simulink model "WCS_Simulink"  (Simulink 8.1)
settings: Solver=ode4  StartTime=0.0  StopTime=Tf  FixedStep=delta_t  RelTol=1e-3
values from neighbouring files (symbols this model uses):
  A = [-3 0;0 0.2]    [Linear_WCS_main.m]
  B = [1; 1]    [Linear_WCS_main.m]
  C = [1 1]    [Linear_WCS_main.m]
  delta_t = 1/sensor_sampling_rate    (= 0.2)    [Linear_WCS_main.m]
  T = [1 1;0 1]    [Linear_WCS_main.m]
  uini = 0    [Linear_WCS_main.m]
  Xini = [x1ini;x2ini]    [Linear_WCS_main.m]
  Xsp = [x1sp;x2sp]    [Linear_WCS_main.m]
settings Model: Creator=Rhine  LastModifiedBy=yehanspc

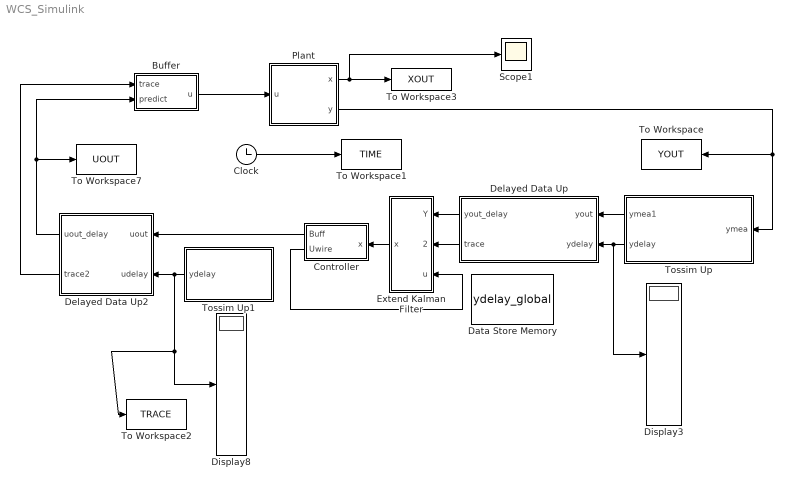
== system WCS_Simulink ==
  Buffer : Subsystem
  Clock : Clock
  Controller : Subsystem
  Data Store Memory : DataStoreMemory  DataStoreName=ydelay_global  ReadBeforeWriteMsg=warning  WriteAfterWriteMsg=warning  WriteAfterReadMsg=warning  InitialValue=[1; 1; 1; 1; 1; 1; 1; 1; 1; 1; 1; 1; 1; 1; 1]  OutDataTypeStr=uint32
  Delayed Data Up : MATLAB Function  TreatAsAtomicUnit=on
  Delayed Data Up2 : MATLAB Function  TreatAsAtomicUnit=on
  Display3 : Display
  Display8 : Display
  Extend Kalman Filter : Subsystem
  Plant : Subsystem
  Scope1 : Scope
  To Workspace : ToWorkspace  VariableName=YOUT  SampleTime=-1
  To Workspace1 : ToWorkspace  VariableName=TIME  SampleTime=-1
  To Workspace2 : ToWorkspace  VariableName=TRACE  SampleTime=-1
  To Workspace3 : ToWorkspace  VariableName=XOUT  SampleTime=-1
  To Workspace7 : ToWorkspace  VariableName=UOUT  SampleTime=-1
  Tossim Up : MATLAB Function  TreatAsAtomicUnit=on
  Tossim Up1 : MATLAB Function  TreatAsAtomicUnit=on
  wires:
  Clock/1 -> To Workspace1/1
  Tossim Up/1(ymea1) -> Delayed Data Up/1(yout)
  Tossim Up/2(ydelay) -> Display3/1, Delayed Data Up/2(ydelay)
  Plant/2(y) -> Tossim Up/1(ymea), To Workspace/1
  Tossim Up1/1(ydelay) -> Delayed Data Up2/2(udelay), To Workspace2/1, Display8/1
  Controller/2(Uwire) -> Extend Kalman Filter/3(u)
  Delayed Data Up/1(yout_delay) -> Extend Kalman Filter/1(Y)
  Extend Kalman Filter/1(x) -> Controller/1(x)
  Plant/1(x) -> Scope1/1, To Workspace3/1
  Delayed Data Up/2(trace) -> Extend Kalman Filter/2("trace ")
  Delayed Data Up2/2(trace2) -> Buffer/1(trace)
  Delayed Data Up2/1(uout_delay) -> Buffer/2(predict), To Workspace7/1
  Controller/1(Buff) -> Delayed Data Up2/1(uout)
  Buffer/1(u) -> Plant/1(u)

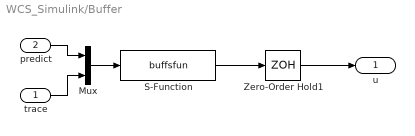
== system WCS_Simulink/Buffer ==
  trace : Inport
  predict : Inport  Port=2
  Mux : Mux  Inputs=2
  S-Function : S-Function  FunctionName=buffsfun  EnableBusSupport=off
  Zero-Order Hold1 : ZeroOrderHold  SampleTime=delta_t
  u : Outport
  wires:
  S-Function/1 -> Zero-Order Hold1/1
  Zero-Order Hold1/1 -> u/1
  Mux/1 -> S-Function/1
  predict/1 -> Mux/1
  trace/1 -> Mux/2

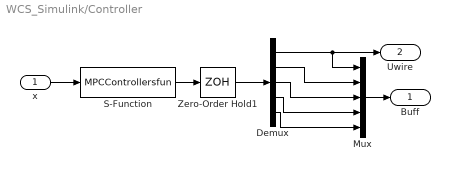
== system WCS_Simulink/Controller ==
  x : Inport
  Demux : Demux  Outputs=5
  Mux : Mux  Inputs=5
  S-Function : S-Function  FunctionName=MPCControllersfun  Parameters=A,B,C,T,uini,Xsp,delta_t  EnableBusSupport=off
  Zero-Order Hold1 : ZeroOrderHold  SampleTime=delta_t
  Buff : Outport
  Uwire : Outport  Port=2
  wires:
  x/1 -> S-Function/1
  S-Function/1 -> Zero-Order Hold1/1
  Zero-Order Hold1/1 -> Demux/1
  Demux/1 -> Mux/1, Uwire/1
  Mux/1 -> Buff/1
  Demux/2 -> Mux/2
  Demux/3 -> Mux/3
  Demux/4 -> Mux/4
  Demux/5 -> Mux/5

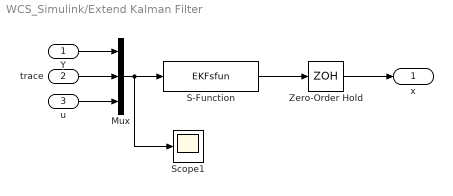
== system WCS_Simulink/Extend Kalman Filter ==
  Y : Inport
  "trace " : Inport  Port=2
  u : Inport  Port=3
  Mux : Mux  Inputs=3
  S-Function : S-Function  FunctionName=EKFsfun  Parameters=A,B,C,T,delta_t  EnableBusSupport=off
  Scope1 : Scope
      settings: SaveName=ScopeData2
  Zero-Order Hold : ZeroOrderHold  SampleTime=delta_t
  x : Outport
  wires:
  Y/1 -> Mux/1
  Mux/1 -> Scope1/1, S-Function/1
  u/1 -> Mux/3
  S-Function/1 -> Zero-Order Hold/1
  Zero-Order Hold/1 -> x/1
  "trace "/1 -> Mux/2

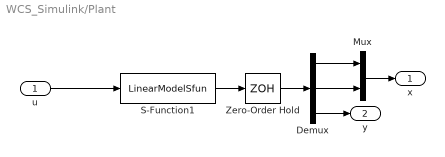
== system WCS_Simulink/Plant ==
  u : Inport
  Demux : Demux  Outputs=3
  Mux : Mux  Inputs=2
  S-Function1 : S-Function  FunctionName=LinearModelSfun  Parameters=A,B,C,T,Xini  EnableBusSupport=off
  Zero-Order Hold : ZeroOrderHold  SampleTime=delta_t
  x : Outport
  y : Outport  Port=2
  wires:
  S-Function1/1 -> Zero-Order Hold/1
  u/1 -> S-Function1/1
  Zero-Order Hold/1 -> Demux/1
  Demux/1 -> Mux/1
  Demux/2 -> Mux/2
  Mux/1 -> x/1
  Demux/3 -> y/1

== matlab function Tossim Up ==
  data: ymea1 output double; ymea input double; ydelay output double; ydelay_global data_store_memory double
function [ymea1, ydelay]  = Tossim_block(ymea)
% Inputs:
% ymea: measurement from structure
% Outputs:
% ymea1: measurement output
% ydelay: delay traces
persistent delay1 % delay trace
persistent i  % count
global ydelay_global


% allow these matlab functions to be used in Embedded Matlab block
eml.extrinsic('python');
eml.extrinsic('num2str');
eml.extrinsic('str2num');
eml.extrinsic('delay_summary');
eml.extrinsic('disp');
eml.extrinsic('ps_aggregation');
eml.extrinsic('for');
eml.extrinsic('end');

if isempty(i)
    i = 0;
end

ydelay = [1 0 0 0 0 0 0 0 0]';
% call python to communicate with TOSSIM

call_count = 18; %Superframelength
rssi = -69;%sensor rssi

[resultz] = ps_aggregation(call_count, rssi);%here call TOSSIM Client ----yh
end_to_end_delivery_result_aggregated = sum(resultz)

resultz

[delay] = delay_summary(end_to_end_delivery_result_aggregated);

delay

ydelay = delay';

delay1 = ydelay;
x =ydelay(2);
i = i+1;

ymea1 = ymea;

for i_yg = 1:9
    ydelay_global(i_yg, 1) = ydelay(i_yg, 1);
end

== matlab function Delayed Data Up ==
  data: yout input double; ydelay input double; yout_delay output double; structure parameter double; trace output double
function [yout_delay,trace]   = delay_block(yout,ydelay, structure)

% Inputs: 
% yout: measurements output
% ydelay: delay traces
% structure: other necessary information 
% Inputs: 
% yout: measurements output
% ydelay: delay traces
% Outputs:
% yout_delay: delayed measurements output for controller

persistent  i yin_d 
persistent yin delay yin_all num
eml.extrinsic('disp');

step_count=100000; %step_count

% initialize parameters
if isempty(yin)
    i = structure.i;
    yin = structure.yin; 
    yin_all = zeros(step_count+1,1); %zeros (step count, sensor number)    
    num = 0;
end

num = num+1;   

%get delay information 
delay=ydelay';

%get value from "yout" input
for kk = 1:1
    yin_all(num,kk) = yout(kk);
end    
    
%generate output value according to delay    
for j=2:2
    if delay(1,j+1)~=88
        yin = yin_all(num,1);  %packet receive
        traces=1;
    else
        yin=0;
        traces=0;        
    end
end

yin_d = yin';
yout_delay = yin_d;
trace=traces;

i = i+1;

== matlab function Delayed Data Up2 ==
  data: uout input double; uout_delay output double; udelay input double; trace2 output double
function [uout_delay,trace2]   = delay_blocku(uout,udelay)

% Inputs: 
% yout: measurements output
% udelay: delay traces
% structure: other necessary information 
% Inputs: 
% yout: measurements output
% udelay: delay traces
% Outputs:
% yout_delay: delayed measurements output for controller

 delay = udelay';

 for j=1
     if delay(1,j+1)~=88
         uoutt_delay=uout;
         tracea=1;
     else
         uoutt_delay=zeros(5,1);
                tracea=0;
     end
 end

 uout_delay=uoutt_delay;
 trace2=tracea;

== matlab function Tossim Up1 ==
  data: ydelay output double; ydelay_global data_store_memory double
function ydelay   = Tossim_block
% ydelay: delay traces
persistent i  % count

% allow these matlab functions to be used in Embedded Matlab block
eml.extrinsic('python');
eml.extrinsic('num2str');
eml.extrinsic('delay_summary');
eml.extrinsic('disp');
if isempty(i)
    i = 0;
end

ydelay = ones (9, 1);

global ydelay_global
for i_tb1 = 1:9
    ydelay(i_tb1, 1) = ydelay_global(i_tb1, 1);
end

i = i+1;
